simulink model "taskBasedWalking_legacy"  (Simulink 8.3)
settings: Solver=FixedStepDiscrete  StartTime=0.0  StopTime=Config.t_end  FixedStep=Config.t_step  RelTol=1e-3
InitFcn:
  | cd(fileparts(which(bdroot)));
  | initTaskBasedWalking;
StopFcn:
  | cd(fileparts(which(bdroot)));
  | stopTaskBasedWalking;
undefined symbols (not defined in the file): biasVectorConstraint_feet, Config, ConstraintMatrix_feet, DiscIntNeverNeededParam, Gains, ROBOT_DOF, Sat
libraries: WBToolboxLibrary x78
(part 3 of 3)

== system taskBasedWalking_legacy/Robot State and References/Smooth References /Smooth Reference Orientations/Compute Smoothed Ref Orientations ==
  w_R_LFoot_des : Inport
  w_R_RFoot_des : Inport  Port=2
  w_R_rot_task_des : Inport  Port=3
  state : Inport  Port=4
  Compute Rotation Matrix Derivative : MATLAB Function  TreatAsAtomicUnit=on
      settings: PermitHierarchicalResolution=ParametersOnly
  Discrete-Time Integrator1 : DiscreteIntegrator  InitialConditionSource=external  InitialCondition=zeros(3,1)  InitialConditionSetting=State (most efficient)  SampleTime=Config.t_step  ICPrevOutput=DiscIntNeverNeededParam  ICPrevScaledInput=DiscIntNeverNeededParam
  Discrete-Time Integrator2 : DiscreteIntegrator  InitialConditionSource=external  InitialCondition=zeros(3,1)  InitialConditionSetting=State (most efficient)  SampleTime=Config.t_step  ICPrevOutput=DiscIntNeverNeededParam  ICPrevScaledInput=DiscIntNeverNeededParam
  Discrete-Time Integrator5 : DiscreteIntegrator  InitialConditionSource=external  InitialCondition=zeros(3,1)  InitialConditionSetting=State (most efficient)  SampleTime=Config.t_step  ICPrevOutput=DiscIntNeverNeededParam  ICPrevScaledInput=DiscIntNeverNeededParam
  "holder " : WBToolboxLibrary/Utilities/holder 
  holder 1 : WBToolboxLibrary/Utilities/holder 
  holder 2 : WBToolboxLibrary/Utilities/holder 
  w_R_rot_task : Outport
  w_R_RFoot : Outport  Port=2
  w_R_LFoot : Outport  Port=3
  tag scope: w_R_LFoot=global, w_R_LFoot_des=global, w_R_RFoot=global, w_R_RFoot_des=global, w_R_rot_task=global, w_R_rot_task_des=global
  wires:
  "holder "/1 -> Discrete-Time Integrator2/2
  holder 2/1 -> Discrete-Time Integrator5/2
  holder 1/1 -> Discrete-Time Integrator1/2
  Compute Rotation Matrix Derivative/1(RDot_LFoot) -> Discrete-Time Integrator2/1
  Compute Rotation Matrix Derivative/2(RDot_RFoot) -> Discrete-Time Integrator5/1
  Compute Rotation Matrix Derivative/3(RDot_rot_task) -> Discrete-Time Integrator1/1
  Discrete-Time Integrator5/1 -> w_R_RFoot/1, [w_R_RFoot], Compute Rotation Matrix Derivative/5(w_R_RFoot)
  Discrete-Time Integrator1/1 -> [w_R_rot_task], w_R_rot_task/1, Compute Rotation Matrix Derivative/6(w_R_rot_task)
  Discrete-Time Integrator2/1 -> [w_R_LFoot], w_R_LFoot/1, Compute Rotation Matrix Derivative/4(w_R_LFoot)
  w_R_LFoot_des/1 -> Compute Rotation Matrix Derivative/1(w_R_LFoot_des), [w_R_LFoot_des], "holder "/1
  w_R_RFoot_des/1 -> Compute Rotation Matrix Derivative/2(w_R_RFoot_des), [w_R_RFoot_des], holder 2/1
  w_R_rot_task_des/1 -> Compute Rotation Matrix Derivative/3(w_R_rot_task_des), holder 1/1, [w_R_rot_task_des]
  state/1 -> Compute Rotation Matrix Derivative/7(state)

== system taskBasedWalking_legacy/Robot State and References/State Machine/Compute State Velocity/Feet Jacobians ==
  s : Inport
  w_H_b : Inport  Port=2
  Jacobian LFoot : WBToolboxLibrary/wholeBodyModel/Jacobians/Jacobian  frameName=Frames.LEFT_FOOT
  Jacobian RFoot : WBToolboxLibrary/wholeBodyModel/Jacobians/Jacobian  frameName=Frames.RIGHT_FOOT
  J_LFoot : Outport
  J_RFoot : Outport  Port=2
  wires:
  Jacobian LFoot/1 -> J_LFoot/1
  Jacobian RFoot/1 -> J_RFoot/1
  w_H_b/1 -> Jacobian RFoot/1, Jacobian LFoot/1
  s/1 -> Jacobian LFoot/2, Jacobian RFoot/2

== system taskBasedWalking_legacy/Robot State and References/State Machine/Compute Transformation Matrices/Compute Feet to Base Link Transforms ==
  IMU port : Inport
  s : Inport  Port=2
  Constant6 : Constant  Value=eye(4)
  LFoot to base link transform : Subsystem
  LFoot to world transform (fixed base) : WBToolboxLibrary/wholeBodyModel/Kinematics/Forward Kinematics  frameName=Frames.LEFT_FOOT
  RFoot to base link transform : Subsystem
  RFoot to world transform (fixed base) : WBToolboxLibrary/wholeBodyModel/Kinematics/Forward Kinematics  frameName=Frames.RIGHT_FOOT
  b_H_LFoot : Outport
  b_H_RFoot : Outport  Port=2
  wires:
  s/1 -> RFoot to world transform (fixed base)/2, LFoot to world transform (fixed base)/2, RFoot to base link transform/1(s), LFoot to base link transform/1(s)
  Constant6/1 -> LFoot to world transform (fixed base)/1, RFoot to world transform (fixed base)/1
  IMU port/1 -> RFoot to base link transform/2(inertial), LFoot to base link transform/2(inertial)
  LFoot to world transform (fixed base)/1 -> LFoot to base link transform/3(b_H_link)
  RFoot to world transform (fixed base)/1 -> RFoot to base link transform/3(b_H_link)
  RFoot to base link transform/1(b_H_link_corrected) -> b_H_RFoot/1
  LFoot to base link transform/1(b_H_link_corrected) -> b_H_LFoot/1

== system taskBasedWalking_legacy/Robot State and References/State Machine/Compute Transformation Matrices/Compute Fixed Foot to World Transform (MPC) ==
  LFoot_is_fixed (MPC) : Inport
  pos_quat_LFoot (MPC) : Inport  Port=2
  "pos_quat_RFoot (MPC) " : Inport  Port=3
  b_H_LFoot : Inport  Port=4
  b_H_RFoot : Inport  Port=5
  From Position + Quaternion to Transf Matrix : MATLAB Function  TreatAsAtomicUnit=on
      settings: PermitHierarchicalResolution=ParametersOnly
  MATLAB Function : MATLAB Function  TreatAsAtomicUnit=on
      settings: PermitHierarchicalResolution=ParametersOnly
  "holder " : WBToolboxLibrary/Utilities/holder 
  w_walking_H_b_initial : Outport
  w_walking_H_LFoot : Outport  Port=2
  w_walking_H_RFoot : Outport  Port=3
  wires:
  b_H_LFoot/1 -> MATLAB Function/3(b_H_LFoot)
  LFoot_is_fixed (MPC)/1 -> MATLAB Function/5(leftIsFixed)
  From Position + Quaternion to Transf Matrix/1(w_walking_H_LFoot) -> w_walking_H_LFoot/1, MATLAB Function/1(w_H_LFoot)
  From Position + Quaternion to Transf Matrix/2(w_walking_H_RFoot) -> MATLAB Function/2(w_H_RFoot), w_walking_H_RFoot/1
  b_H_RFoot/1 -> MATLAB Function/4(b_H_RFoot)
  MATLAB Function/1(w_H_b) -> "holder "/1
  pos_quat_LFoot (MPC)/1 -> From Position + Quaternion to Transf Matrix/1(qt_LFoot)
  "pos_quat_RFoot (MPC) "/1 -> From Position + Quaternion to Transf Matrix/2(qt_RFoot)
  "holder "/1 -> w_walking_H_b_initial/1

== system taskBasedWalking_legacy/Robot State and References/State Machine/Select Current References and Estimate w_H_b/Emergency Stop ==
  CoM_des : Inport
  Enable : EnablePort
  Constant : Constant  OutDataTypeStr=boolean
  Constant1 : Constant  Value=0  OutDataTypeStr=boolean
  Selector : Selector  InputPortWidth=9  IndexOptions=Index vector (dialog)  Indices=[3]  OutputSizes=1
  Stop Simulation : Stop
  Switch : Switch  Criteria=u2 > Threshold  Threshold=0.1
  holder 1 : WBToolboxLibrary/Utilities/holder 
  wires:
  CoM_des/1 -> Selector/1
  Switch/1 -> Stop Simulation/1
  Constant1/1 -> Switch/1
  Constant/1 -> Switch/3
  Selector/1 -> holder 1/1
  holder 1/1 -> Switch/2

== system taskBasedWalking_legacy/Robot State and References/State Machine/Select Current References and Estimate w_H_b/Smooth the Base Pose and send it to the MPC ==
  w_H_b : Inport
  Constant : Constant  Value=0.01
  Constant1 : Constant  Value=Config.SMOOTH_BASE_POS
  Constant2 : Constant  Value=Config.SMOOTH_BASE_ORIENT
  From Pos Rot to Transf MAtrix : MATLAB Function  TreatAsAtomicUnit=on
      settings: PermitHierarchicalResolution=ParametersOnly
  From Transf Matrix To Position+Quaternion Base : MATLAB Function  TreatAsAtomicUnit=on
      settings: PermitHierarchicalResolution=ParametersOnly
  Minimum Jerk Trajectory Generator : WBToolboxLibrary/Utilities/Minimum Jerk Trajectory Generator  externalSettlingTime=on  settlingTime=3  sampleTime=Config.t_step  resetOnSettlingTime=off  firstDerivatives=on  secondDerivatives=off  explicitInitialValue=off
  Mux : Mux  Inputs=2
  Selector : Selector  NumberOfDimensions=2  InputPortWidth=3  IndexOptions=Index vector (dialog),Index vector (dialog)  Indices=[1:3],4  OutputSizes=1,1
  Selector1 : Selector  NumberOfDimensions=2  InputPortWidth=3  IndexOptions=Index vector (dialog),Index vector (dialog)  Indices=[1:3],[1:3]  OutputSizes=1,1
  Send w_H_b to the planner : WBToolboxLibrary/Utilities/Yarp Write  portName=Ports.BASE_POSE  autoconnect=on  errorOnConnection=off
  Smooth Reference Orientation : Subsystem
  Switch : Switch  Criteria=u2 > Threshold
  Switch1 : Switch  Criteria=u2 > Threshold
  w_H_b_smoothed : Outport
  BaseVelocity : Outport  Port=2
  wires:
  w_H_b/1 -> Selector1/1, Selector/1
  From Pos Rot to Transf MAtrix/1(w_H_b) -> w_H_b_smoothed/1, From Transf Matrix To Position+Quaternion Base/1(w_H_b)
  Constant/1 -> Minimum Jerk Trajectory Generator/2
  Selector/1 -> Switch/3, Minimum Jerk Trajectory Generator/1
  Selector1/1 -> Smooth Reference Orientation/1(w_R_b_des), Switch1/3
  From Transf Matrix To Position+Quaternion Base/1(pos_quat_base) -> Send w_H_b to the planner/1
  Constant1/1 -> Switch/2
  Constant2/1 -> Switch1/2
  Switch/1 -> From Pos Rot to Transf MAtrix/1(pos_b)
  Minimum Jerk Trajectory Generator/1 -> Switch/1
  Switch1/1 -> From Pos Rot to Transf MAtrix/2(w_R_b)
  Smooth Reference Orientation/1(w_R_b) -> Switch1/1
  Minimum Jerk Trajectory Generator/2 -> Mux/1
  Smooth Reference Orientation/2(w_omega) -> Mux/2
  Mux/1 -> BaseVelocity/1

== system taskBasedWalking_legacy/Robot State and References/State Machine/Compute Transformation Matrices/Compute Feet to Base Link Transforms/LFoot to base link transform ==
  s : Inport
  inertial : Inport  Port=2
  b_H_link : Inport  Port=3
  Constant6 : Constant  Value=eye(4)
  Fixed base to imu transform : WBToolboxLibrary/wholeBodyModel/Kinematics/Forward Kinematics  frameName=Frames.IMU
  Inv\* : Product  Inputs=/*  Multiplication=Matrix(*)
  "Inv\\*  " : Product  Inputs=/  Multiplication=Matrix(*)
  Inv\*  1 : Product  Inputs=/  Multiplication=Matrix(*)
  Neck Position : WBToolboxLibrary/Utilities/Yarp Read  portName=Ports.NECK_POS  signalSize=6  timeout=0.5  blocking=off  timestamp=off  autoconnect=on  errorOnConnection=off
  Switch6 : Switch  Criteria=u2 > Threshold
  USE_IMU4EST_BASE : Constant  Value=Config.USE_IMU4EST_BASE
  fromImuToHomogeousTransformFCN : MATLAB Function  TreatAsAtomicUnit=on
      settings: PermitHierarchicalResolution=ParametersOnly
  holder 1 : WBToolboxLibrary/Utilities/holder 
  holder 2 : WBToolboxLibrary/Utilities/holder 
  neck transform : Subsystem
  b_H_link_corrected : Outport
  wires:
  Switch6/1 -> b_H_link_corrected/1
  "Inv\\*  "/1 -> fromImuToHomogeousTransformFCN/3(link_H_base)  "link_H_b"
  USE_IMU4EST_BASE/1 -> Switch6/2
  Inv\*/1 -> fromImuToHomogeousTransformFCN/1(imu_H_link), holder 1/1  "imu_H_link"
  holder 2/1 -> fromImuToHomogeousTransformFCN/4(inertial_0)
  Fixed base to imu transform/1 -> Inv\*/1
  holder 1/1 -> fromImuToHomogeousTransformFCN/2(imu_H_link_0)
  s/1 -> Fixed base to imu transform/2
  fromImuToHomogeousTransformFCN/1(w_H_b) -> Inv\*  1/1
  inertial/1 -> holder 2/1, fromImuToHomogeousTransformFCN/5(inertial)
  Neck Position/1 -> neck transform/1(neck port)
  neck transform/1(neck position) -> fromImuToHomogeousTransformFCN/6(neck_pos)
  b_H_link/1 -> Switch6/3, "Inv\\*  "/1, Inv\*/2
  Constant6/1 -> Fixed base to imu transform/1
  Inv\*  1/1 -> Switch6/1

== system taskBasedWalking_legacy/Robot State and References/State Machine/Compute Transformation Matrices/Compute Feet to Base Link Transforms/RFoot to base link transform ==
  s : Inport
  inertial : Inport  Port=2
  b_H_link : Inport  Port=3
  Constant6 : Constant  Value=eye(4)
  Fixed base to imu transform : WBToolboxLibrary/wholeBodyModel/Kinematics/Forward Kinematics  frameName=Frames.IMU
  Inv\* : Product  Inputs=/*  Multiplication=Matrix(*)
  "Inv\\*  " : Product  Inputs=/  Multiplication=Matrix(*)
  Inv\*  1 : Product  Inputs=/  Multiplication=Matrix(*)
  Neck Position : WBToolboxLibrary/Utilities/Yarp Read  portName=Ports.NECK_POS  signalSize=6  timeout=0.5  blocking=off  timestamp=off  autoconnect=on  errorOnConnection=off
  Switch6 : Switch  Criteria=u2 > Threshold
  USE_IMU4EST_BASE : Constant  Value=Config.USE_IMU4EST_BASE
  fromImuToHomogeousTransformFCN : MATLAB Function  TreatAsAtomicUnit=on
      settings: PermitHierarchicalResolution=ParametersOnly
  holder 1 : WBToolboxLibrary/Utilities/holder 
  holder 2 : WBToolboxLibrary/Utilities/holder 
  neck transform : Subsystem
  b_H_link_corrected : Outport
  wires:
  Switch6/1 -> b_H_link_corrected/1
  "Inv\\*  "/1 -> fromImuToHomogeousTransformFCN/3(link_H_base)  "link_H_b"
  USE_IMU4EST_BASE/1 -> Switch6/2
  Inv\*/1 -> fromImuToHomogeousTransformFCN/1(imu_H_link), holder 1/1  "imu_H_link"
  holder 2/1 -> fromImuToHomogeousTransformFCN/4(inertial_0)
  Fixed base to imu transform/1 -> Inv\*/1
  holder 1/1 -> fromImuToHomogeousTransformFCN/2(imu_H_link_0)
  s/1 -> Fixed base to imu transform/2
  fromImuToHomogeousTransformFCN/1(w_H_b) -> Inv\*  1/1
  inertial/1 -> holder 2/1, fromImuToHomogeousTransformFCN/5(inertial)
  Neck Position/1 -> neck transform/1(neck port)
  neck transform/1(neck position) -> fromImuToHomogeousTransformFCN/6(neck_pos)
  b_H_link/1 -> Switch6/3, "Inv\\*  "/1, Inv\*/2
  Constant6/1 -> Fixed base to imu transform/1
  Inv\*  1/1 -> Switch6/1

== system taskBasedWalking_legacy/Robot State and References/State Machine/Select Current References and Estimate w_H_b/Smooth the Base Pose and send it to the MPC/Smooth Reference Orientation ==
  w_R_b_des : Inport
  Compute Rotation Matrix Derivative : MATLAB Function  TreatAsAtomicUnit=on
      settings: PermitHierarchicalResolution=ParametersOnly
  Discrete-Time Integrator : DiscreteIntegrator  InitialConditionSource=external  InitialCondition=zeros(3,1)  InitialConditionSetting=State (most efficient)  SampleTime=Config.t_step  ICPrevOutput=DiscIntNeverNeededParam  ICPrevScaledInput=DiscIntNeverNeededParam
  "holder " : WBToolboxLibrary/Utilities/holder 
  w_R_b : Outport
  w_omega : Outport  Port=2
  tag scope: VDot_base=global, V_base=global
  wires:
  Discrete-Time Integrator/1 -> w_R_b/1, Compute Rotation Matrix Derivative/1(w_R_b)
  w_R_b_des/1 -> "holder "/1, Compute Rotation Matrix Derivative/2(w_R_b_des)
  Compute Rotation Matrix Derivative/1(w_RDot_b) -> Discrete-Time Integrator/1
  "holder "/1 -> Discrete-Time Integrator/2
  Compute Rotation Matrix Derivative/3(V) -> [V_base]
  Compute Rotation Matrix Derivative/4(VDot) -> [VDot_base]
  Compute Rotation Matrix Derivative/2(w_omega) -> w_omega/1

== system taskBasedWalking_legacy/Robot State and References/State Machine/Compute Transformation Matrices/Compute Feet to Base Link Transforms/LFoot to base link transform/neck transform ==
  neck port : Inport
  Constant : Constant  Value=zeros(3,1)
  Gain : Gain  Gain=pi/180
  Selector1 : Selector  InputPortWidth=6  IndexOptions=Index vector (dialog)  Indices=[1:3]  OutputSizes=1
  Switch : Switch  Criteria=u2 > Threshold
  USE_IMU4EST_BASE1 : Constant  Value=Config.CORRECT_IMU_WITH_NECK_POS
  neck position : Outport
  wires:
  neck port/1 -> Gain/1
  USE_IMU4EST_BASE1/1 -> Switch/2
  Switch/1 -> neck position/1
  Gain/1 -> Selector1/1
  Constant/1 -> Switch/3
  Selector1/1 -> Switch/1  "neck pos"

== system taskBasedWalking_legacy/Robot State and References/State Machine/Compute Transformation Matrices/Compute Feet to Base Link Transforms/RFoot to base link transform/neck transform ==
  neck port : Inport
  Constant : Constant  Value=zeros(3,1)
  Gain : Gain  Gain=pi/180
  Selector1 : Selector  InputPortWidth=6  IndexOptions=Index vector (dialog)  Indices=[1:3]  OutputSizes=1
  Switch : Switch  Criteria=u2 > Threshold
  USE_IMU4EST_BASE1 : Constant  Value=Config.CORRECT_IMU_WITH_NECK_POS
  neck position : Outport
  wires:
  neck port/1 -> Gain/1
  USE_IMU4EST_BASE1/1 -> Switch/2
  Switch/1 -> neck position/1
  Gain/1 -> Selector1/1
  Constant/1 -> Switch/3
  Selector1/1 -> Switch/1  "neck pos"

== matlab function Visualization/Visualize Joints and Floating Base State/Rotation Error Base1/Rot error using roll-pitch-yaw ==
  data: R_0 input double; rollPitchYaw output double
function rollPitchYaw = rollPitchYawFromRotationFCN(R_0)

    rollPitchYaw = rollPitchYawFromRotation(R_0);
end

== matlab function Balancing Controller (Reactive QP control)/Balancing Controller Function ==
  data: feetInContact input double; M input double; Hessian output double; h input double; J input double; impedances input double; dampings input double; s input double; sDot input double; s_sDot_sDDot_des input double; acc_task_star input double; JDot_nu input double; ConstraintsMatrix_feet input double; biasVectorConstraint_feet input double; w_H_l_sole input double; w_H_r_sole input double; gradient output double; ConstraintMatrix_equality output double; biasVectorConstraint_equality output double; ConstraintMatrix_inequality output double; biasVectorConstraint_inequality output double; Sat parameter double; weightsForces input double; leftIsFixed input double
function [Hessian,gradient,ConstraintMatrix_equality,biasVectorConstraint_equality, ...
          ConstraintMatrix_inequality,biasVectorConstraint_inequality] = ...
          balancingControllerFCN(feetInContact, M, h, J, impedances, ...
                                 dampings, s, sDot, s_sDot_sDDot_des, acc_task_star, ...
                                 JDot_nu, ConstraintsMatrix_feet, biasVectorConstraint_feet, ...
                                 w_H_l_sole, w_H_r_sole, Sat, weightsForces, leftIsFixed)
                          

    [Hessian,gradient,ConstraintMatrix_equality,biasVectorConstraint_equality, ...
     ConstraintMatrix_inequality,biasVectorConstraint_inequality] = ...
         balancingControllerMPC(feetInContact, M, h, J, impedances, ...
                                dampings, s, sDot, s_sDot_sDDot_des, acc_task_star, ...
                                JDot_nu, ConstraintsMatrix_feet, biasVectorConstraint_feet, ...
                                w_H_l_sole, w_H_r_sole, Sat, weightsForces, leftIsFixed);                         
end

== matlab function Dynamics and Kinematics/Compute Tasks Accelerations/Compute tasks accelerations ==
  data: pos_vel_acc_CoM_des input double; acc_task_star output double; pose_vel_acc_LFoot_des input double; pose_vel_acc_RFoot_des input double; orient_vel_acc_rot_task_des input double; pos_vel_CoM input double; pose_vel_LFoot input double; pose_vel_RFoot input double; orient_vel_rot_task input double; Kp_Kd_CoM input double; Kp_Kd_LFoot input double; Kp_Kd_RFoot input double; Kp_Kd_rot_task input double; feetInContact input double; useFeetPIDs input double; Sat parameter double; Config parameter double
function acc_task_star = setTasksAccelerationsFCN(pos_vel_acc_CoM_des,pose_vel_acc_LFoot_des,pose_vel_acc_RFoot_des,orient_vel_acc_rot_task_des, ...
                                                  pos_vel_CoM, pose_vel_LFoot, pose_vel_RFoot, orient_vel_rot_task, ...
                                                  Kp_Kd_CoM, Kp_Kd_LFoot, Kp_Kd_RFoot, Kp_Kd_rot_task, feetInContact, useFeetPIDs, Sat, Config) 

    acc_task_star = setTasksAccelerations(pos_vel_acc_CoM_des,pose_vel_acc_LFoot_des,pose_vel_acc_RFoot_des,orient_vel_acc_rot_task_des, ...
                                          pos_vel_CoM, pose_vel_LFoot, pose_vel_RFoot, orient_vel_rot_task, ...
                                          Kp_Kd_CoM, Kp_Kd_LFoot, Kp_Kd_RFoot, Kp_Kd_rot_task, feetInContact, useFeetPIDs, Sat, Config); 
end

== matlab function Dynamics and Kinematics/Compute Tasks Accelerations/ComputeTasksPoseAndVelocity/Compose Task Pose and Velocity ==
  data: vel_CoM input double; vel_LFoot input double; vel_RFoot input double; vel_rot_task input double; pos_vel_CoM output double; pose_vel_LFoot output double; pose_vel_RFoot output double; orient_vel_rot_task output double; w_H_CoM input double; w_H_l_sole input double; w_H_r_sole input double; w_H_rot_task input double
function [pos_vel_CoM, pose_vel_LFoot, pose_vel_RFoot, orient_vel_rot_task] = ...
             composeTaskPoseAndVelocityFCN(vel_CoM, vel_LFoot, vel_RFoot, vel_rot_task, ...
                                           w_H_CoM, w_H_l_sole, w_H_r_sole, w_H_rot_task)
                                                                                                                              
    [pos_vel_CoM, pose_vel_LFoot, pose_vel_RFoot, orient_vel_rot_task] = ...
        composeTaskPoseAndVelocity(vel_CoM, vel_LFoot, vel_RFoot, vel_rot_task, ...
                                   w_H_CoM, w_H_l_sole, w_H_r_sole, w_H_rot_task);
end

== matlab function Robot State and References/Gain Scheduling/Gain Scheduling Function ==
  data: state input double; Kp_CoM output double; Kd_CoM output double; Kp_LFoot output double; Kd_LFoot output double; Kp_RFoot output double; Kd_RFoot output double; Kp_rot_task output double; Kd_rot_task output double; impedances output double; dampings output double; Gains parameter double; smoothingTimeGains output double; Config parameter double
function [Kp_CoM, Kd_CoM, Kp_LFoot, Kd_LFoot, Kp_RFoot, Kd_RFoot, Kp_rot_task, Kd_rot_task, impedances, dampings, smoothingTimeGains] = ...
             gainSchedulingFCN(state,Gains,Config)

    [Kp_CoM, Kd_CoM, Kp_LFoot, Kd_LFoot, Kp_RFoot, Kd_RFoot, Kp_rot_task, Kd_rot_task, impedances, dampings, smoothingTimeGains] = ...
        gainScheduling(state,Gains,Config);
end

== matlab function Robot State and References/State Machine/Select Current References and Estimate w_H_b/STATE MACHINES ==
  data: s_0 input double; w_H_rot_task_initial input double; w_walking_H_LFoot input double; w_walking_H_RFoot input double; b_H_LFoot input double; b_H_RFoot input double; b_H_RFoot_desired input double; LFoot_is_fixed input double; pos_vel_acc_CoM_des_walking input double; s_des_walking input double; feetInContact_walking input double; LFoot_wrench input double; RFoot_wrench input double; waistImu input double; state output double; references_CoM output double; references_LFoot output double; references_RFoot output double; references_rot_task output double; feetInContact output double; references_s output double; w_H_b output double; w_H_bWithImu output double; Config parameter double; leftIsFixed_out output double; useFeetPIDs output double; Sat parameter double; omega_world output double
function [state, references_CoM, references_LFoot, references_RFoot, references_rot_task, feetInContact, references_s, w_H_b, w_H_bWithImu, leftIsFixed_out, useFeetPIDs, omega_world] = stateMachinesFCN ...
             (s_0, w_H_rot_task_initial, w_walking_H_LFoot, w_walking_H_RFoot, b_H_LFoot, b_H_RFoot, b_H_RFoot_desired, LFoot_is_fixed, pos_vel_acc_CoM_des_walking, ...
              s_des_walking, feetInContact_walking, LFoot_wrench, RFoot_wrench, waistImu, Config, Sat)
        
        % Footstep planner + MPC State Machine
        [state, references_CoM, references_LFoot, references_RFoot, references_rot_task, feetInContact, references_s, w_H_b, w_H_bWithImu, leftIsFixed_out, useFeetPIDs, omega_world] = stateMachineWalking ...
            (s_0, pos_vel_acc_CoM_des_walking, s_des_walking, feetInContact_walking, b_H_LFoot, b_H_RFoot, w_walking_H_LFoot, w_walking_H_RFoot, w_H_rot_task_initial, ...
             b_H_RFoot_desired, LFoot_is_fixed, LFoot_wrench, RFoot_wrench, waistImu, Config, Sat); 
end

== matlab function Robot State and References/State Machine/Select Current References and Estimate w_H_b/Smooth the Base Pose and send it to the MPC/From Transf Matrix To Position+Quaternion Base ==
  data: w_H_b input double; pos_quat_base output double
function pos_quat_base = fromTransfMatrixToPosQuatFCN(w_H_b) 

    pos_quat_base = fromTransfMatrixToPosQuat(w_H_b); 
end

== matlab function Robot State and References/Smooth References /Smooth Reference Orientations/Compute Smoothed Ref Orientations/Compute Rotation Matrix Derivative ==
  data: RDot_LFoot output double; RDot_RFoot output double; RDot_rot_task output double; w_R_LFoot_des input double; w_R_RFoot_des input double; w_R_rot_task_des input double; w_R_LFoot input double; w_R_RFoot input double; w_R_rot_task input double; state input double; Config parameter double
function [RDot_LFoot, RDot_RFoot, RDot_rot_task] = rotationDerivativeFromAngVelFCN(w_R_LFoot_des, w_R_RFoot_des, w_R_rot_task_des, ... 
                                                                                   w_R_LFoot, w_R_RFoot, w_R_rot_task, state, Config)
      
                                                                                                                                                         
    % Compute the input angular velocity (expressed in world frame)
    
    % Left foot
    w_omegaLFoot_des     = zeros(3,1);
    Kp_LFoot             = Config.LFoot_Kp_smoothing(state);
    w_omegaLFoot         = rotationalPID_velocity(w_R_LFoot,w_R_LFoot_des,w_omegaLFoot_des,Kp_LFoot);
    
    % Right foot
    w_omegaRFoot_des     = zeros(3,1);
    Kp_RFoot             = Config.RFoot_Kp_smoothing(state);
    w_omegaRFoot         = rotationalPID_velocity(w_R_RFoot,w_R_RFoot_des,w_omegaRFoot_des,Kp_RFoot);
    
    % Rot task
    w_omega_rot_task_des = zeros(3,1);
    Kp_rot_task          = Config.rot_task_Kp_smoothing(state);
    w_omega_rot_task     = rotationalPID_velocity(w_R_rot_task,w_R_rot_task_des,w_omega_rot_task_des,Kp_rot_task);
                                    
    % Compute the rotation matrix derivative given the angular velocity
    RDot_LFoot     = rotationDerivativeFromAngVel(w_omegaLFoot,w_R_LFoot);
    RDot_RFoot     = rotationDerivativeFromAngVel(w_omegaRFoot,w_R_RFoot);
    RDot_rot_task  = rotationDerivativeFromAngVel(w_omega_rot_task, w_R_rot_task);      
end

== matlab function Robot State and References/State Machine/Compute Transformation Matrices/Compute Feet to Base Link Transforms/RFoot to base link transform/fromImuToHomogeousTransformFCN ==
  data: imu_H_link input double; imu_H_link_0 input double; link_H_base input double; inertial_0 input double; inertial input double; neck_pos input double; w_H_b output double; Config parameter double
function w_H_b = worldToBaseTransformWithIMUFCN(imu_H_link,imu_H_link_0,link_H_base,inertial_0,inertial,neck_pos,Config)

    w_H_b = worldToBaseTransformWithIMU(imu_H_link,imu_H_link_0,link_H_base,inertial_0,inertial,neck_pos,Config);

end

== matlab function Robot State and References/State Machine/Compute State Velocity/Compute Base Velocity ==
  data: J_LeftFoot input double; J_RightFoot input double; feetInContact input double; nu_b output double; sDot input double; Sat parameter double
function nu_b = computeBaseVelocityFCN(J_LeftFoot,J_RightFoot, feetInContact, sDot, Sat)

    nu_b = computeBaseVelocity(J_LeftFoot,J_RightFoot, feetInContact, sDot, Sat);
end

== matlab function Robot State and References/Smooth References /Smooth Reference Positions/Configure Settling Times ==
  data: state input double; Config parameter double; smoothingTime_CoM output double; smoothingTime_joints output double; smoothingTime_LFoot output double; smoothingTime_RFoot output double
function [smoothingTime_CoM, smoothingTime_joints, smoothingTime_LFoot, smoothingTime_RFoot] = setSmoothingTimesFCN(state,Config)

    [smoothingTime_CoM, smoothingTime_LFoot, smoothingTime_RFoot, smoothingTime_joints] = setSmoothingTimes(state,Config);

end

== matlab function Dynamics and Kinematics/Compute Dynamic and Kinematic Quantities/Mass Matrix and Bias Forces/Add motors reflected inertias/Add motor reflected inertias ==
  data: M input double; M_with_inertia output double; Config parameter double
function M_with_inertia = addMotorsInertiaFCN(M,Config)

    M_with_inertia = addMotorsInertia(M,Config);

end

== matlab function Balancing Controller (Reactive QP control)/Compute joint torques (motor reflected inertia)/(transpose(T*Gamma))^{-1}*I_m*(T*Gamma)^{-1} ==
  data: reflectedInertia output double; Config parameter double
function reflectedInertia  = computeMotorsInertiaFCN(Config)

    [reflectedInertia] = computeMotorsInertia(Config);

end

== matlab function Robot State and References/emergency stop: joint limits/MATLAB Function ==
  data: umin input double; umax input double; u input double; inRange output double; tol input double
function inRange = checkRangeFCN(umin, umax, u, tol)

     inRange = checkRange(umin, umax, u, tol);
end

== matlab function Visualization/Visualize Smoothing (orientation)/Rotation Error Left Foot/Rot error using roll-pitch-yaw ==
  data: R_0 input double; rollPitchYaw output double
function rollPitchYaw = rollPitchYawFromRotationFCN(R_0)

    rollPitchYaw = rollPitchYawFromRotation(R_0);
end

== matlab function Visualization/Visualize Smoothing (orientation)/Rotation Error Right Foot/Rot error using roll-pitch-yaw ==
  data: R_0 input double; rollPitchYaw output double
function rollPitchYaw = rollPitchYawFromRotationFCN(R_0)

    rollPitchYaw = rollPitchYawFromRotation(R_0);
end

== matlab function Robot State and References/State Machine/Compute Transformation Matrices/Compute Fixed Foot to World Transform (MPC)/From Position + Quaternion to Transf Matrix ==
  data: qt_LFoot input double; w_walking_H_LFoot output double; qt_RFoot input double; w_walking_H_RFoot output double
function [w_walking_H_LFoot,w_walking_H_RFoot] = fromPosQuatToTransfMatrFCN(qt_LFoot,qt_RFoot) 

    w_walking_H_LFoot = fromPosQuatToTransfMatr(qt_LFoot); 
    w_walking_H_RFoot = fromPosQuatToTransfMatr(qt_RFoot); 
end

== matlab function Visualization/Visualize Smoothing (orientation)/Rotation Error Rot Task/Rot error using roll-pitch-yaw ==
  data: R_0 input double; rollPitchYaw output double
function rollPitchYaw = rollPitchYawFromRotationFCN(R_0)

    rollPitchYaw = rollPitchYawFromRotation(R_0);
end

== matlab function Robot State and References/State Machine/Compute Transformation Matrices/Compute Fixed Foot to World Transform (MPC)/MATLAB Function ==
  data: w_H_LFoot input double; w_H_b output double; w_H_RFoot input double; b_H_LFoot input double; b_H_RFoot input double; leftIsFixed input double
function w_H_b = getW_H_B(w_H_LFoot, w_H_RFoot, b_H_LFoot, b_H_RFoot, leftIsFixed)

    if round(leftIsFixed) == 1
        w_H_b = w_H_LFoot / b_H_LFoot;
    else
        w_H_b = w_H_RFoot / b_H_RFoot;
    end
end

== matlab function Visualization/Visualize Cartesian Tasks/Rotation Error Left Foot/Rot error using roll-pitch-yaw ==
  data: R_0 input double; rollPitchYaw output double
function rollPitchYaw = rollPitchYawFromRotationFCN(R_0)

    rollPitchYaw = rollPitchYawFromRotation(R_0);
end

== matlab function Robot State and References/State Machine/Select Current References and Estimate w_H_b/Smooth the Base Pose and send it to the MPC/From Pos Rot to Transf MAtrix ==
  data: pos_b input double; w_H_b output double; w_R_b input double
function w_H_b = posRotToTransfMatrixFCN(pos_b, w_R_b) 

    w_H_b = posRotToTransfMatrix(pos_b, w_R_b);
end

== matlab function Visualization/Visualize Cartesian Tasks/Rotation Error Right Foot/Rot error using roll-pitch-yaw ==
  data: R_0 input double; rollPitchYaw output double
function rollPitchYaw = rollPitchYawFromRotationFCN(R_0)

    rollPitchYaw = rollPitchYawFromRotation(R_0);
end

== matlab function Visualization/Visualize Cartesian Tasks/Rotation Error Rot Task/Rot error using roll-pitch-yaw ==
  data: R_0 input double; rollPitchYaw output double
function rollPitchYaw = rollPitchYawFromRotationFCN(R_0)

    rollPitchYaw = rollPitchYawFromRotation(R_0);
end

== matlab function Robot State and References/State Machine/Compute Transformation Matrices/Compute Feet to Base Link Transforms/LFoot to base link transform/fromImuToHomogeousTransformFCN ==
  data: imu_H_link input double; imu_H_link_0 input double; link_H_base input double; inertial_0 input double; inertial input double; neck_pos input double; w_H_b output double; Config parameter double
function w_H_b = worldToBaseTransformWithIMUFCN(imu_H_link,imu_H_link_0,link_H_base,inertial_0,inertial,neck_pos,Config)

    w_H_b = worldToBaseTransformWithIMU(imu_H_link,imu_H_link_0,link_H_base,inertial_0,inertial,neck_pos,Config);

end

== matlab function Robot State and References/State Machine/Select Current References and Estimate w_H_b/Smooth the Base Pose and send it to the MPC/Smooth Reference Orientation/Compute Rotation Matrix Derivative ==
  data: w_R_b input double; w_RDot_b output double; w_omega output double; w_R_b_des input double; Config parameter double; V output double; VDot output double
function [w_RDot_b, w_omega, V,VDot] = rotationDerivativeFromAngVelFCN(w_R_b, w_R_b_des, Config)
    

    % Compute the input angular velocity (expressed in world frame)
    w_omega_des = zeros(3,1);
    Kp          = Config.baseRotation_Kp_smoothing;
    w_omega     = rotationalPID_velocity(w_R_b,w_R_b_des,w_omega_des,Kp);
                                    
    % Compute the rotation matrix derivative given the angular velocity
    w_RDot_b    = rotationDerivativeFromAngVel(w_omega,w_R_b);
    
    %% Debug: Lyapunov Function and its derivative
    V    = trace(eye(3)-w_R_b*transpose(w_R_b_des));
    VDot = transpose(w_omega-w_omega_des)*skewVee(w_R_b*transpose(w_R_b_des));
end

== matlab function Visualization/Visualize Joints and Floating Base State/Rotation Error Base/Rot error using roll-pitch-yaw ==
  data: R_0 input double; rollPitchYaw output double
function rollPitchYaw = rollPitchYawFromRotationFCN(R_0)

    rollPitchYaw = rollPitchYawFromRotation(R_0);
end
